simulink model "ModeloSimulink"  (R2021b)
settings: Solver=VariableStepAuto  StartTime=0.0  StopTime=3  MaxStep=1e-3  RelTol=1e-3
libraries: simulink x1
settings Model: Creator=carlo  LastModifiedBy=carlo
settings SolverCC: AlgebraicLoopSolver=TrustRegion
settings DebuggingCC: SFMachineParentedDataDiag=warning

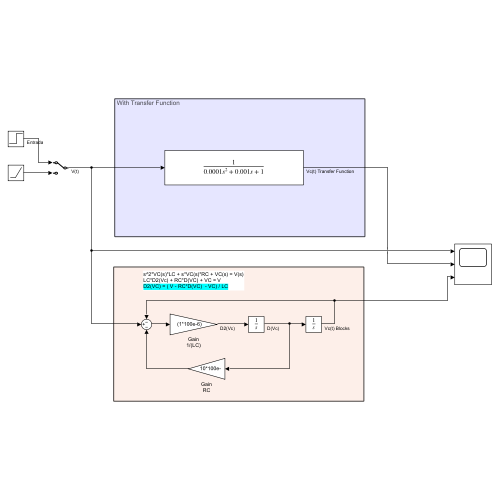
[thumbnail: Simulink's stored preview of the top-level diagram]
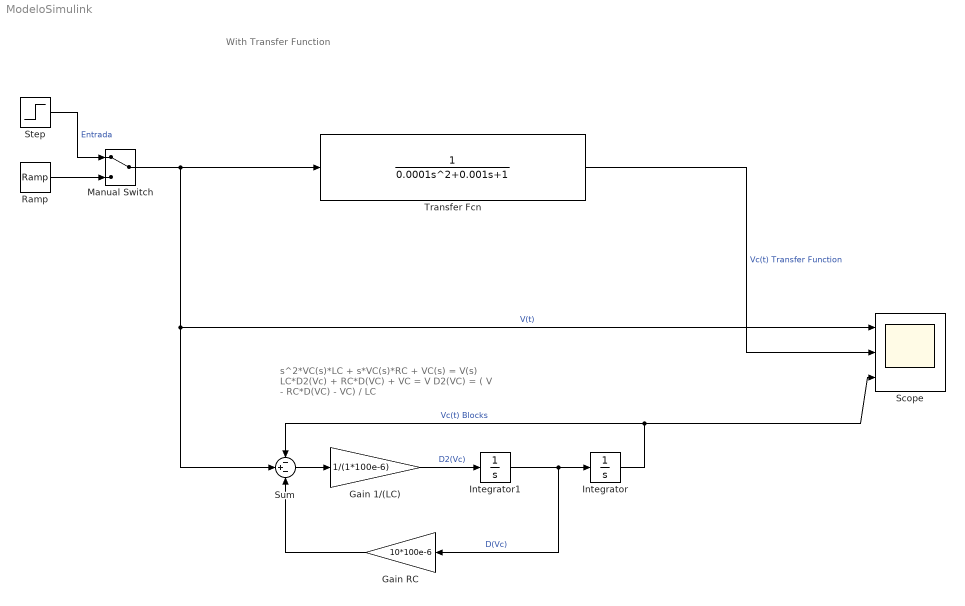
== system ModeloSimulink ==
  note: s^2*VC(s)*LC + s*VC(s)*RC + VC(s) = V(s)
      | LC*D2(Vc) + RC*D(VC) + VC = V
      | D2(VC) = ( V - RC*D(VC) - VC) / LC
  note: With Transfer Function
  Gain 1/(LC) : Gain  Gain=1/(1*100e-6)
  Gain RC : Gain  Gain=10*100e-6
  Integrator : Integrator  InitialCondition=8
  Integrator1 : Integrator
  Manual Switch : ManualSwitch
  Ramp : simulink/Sources/Ramp  slope=1  start=1  InitialOutput=0
  Scope : Scope  NumInputPorts=3
  Step : Step  Time=0  After=12  SampleTime=0
  Sum : Sum  Inputs=-+-
  Transfer Fcn : TransferFcn  Denominator=[0.0001 0.001 1]
  wires:
  Step/1 -> Manual Switch/1  "Entrada"
  Ramp/1 -> Manual Switch/2
  Manual Switch/1 -> Sum/2, Scope/1, Transfer Fcn/1  "V(t)"
  Integrator1/1 -> Gain RC/1, Integrator/1  "D(Vc)"
  Gain 1/(LC)/1 -> Integrator1/1  "D2(Vc)"
  Sum/1 -> Gain 1/(LC)/1
  Transfer Fcn/1 -> Scope/2  "Vc(t) Transfer Function"
  Integrator/1 -> Scope/3, Sum/1  "Vc(t) Blocks"
  Gain RC/1 -> Sum/3
